simulink library "modularPlant_cl"  (R2018b)
settings: Solver=VariableStepAuto  StartTime=0.0  StopTime=10.0  RelTol=1e-3
undefined symbols (not defined in the file or in its folder): sim_param
libraries: animation_cl x1, fixedGroundStation_cl x1, tethers_cl x1, vehicle x1, winch_ul x1
settings Model: Creator=mcobb  LastModifiedBy=mcobb

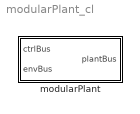
== system modularPlant_cl ==
  modularPlant : Subsystem  VariantControl=VSS_plant_modularPlant

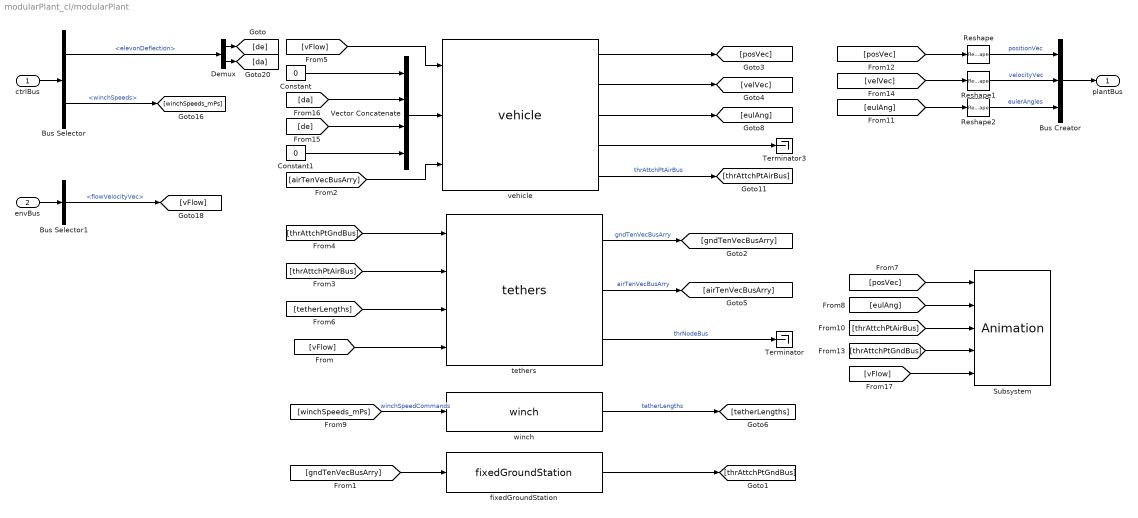
== system modularPlant_cl/modularPlant ==
  ctrlBus : Inport  OutDataTypeStr=Bus: ctrlBus
  envBus : Inport  Port=2  OutDataTypeStr=Bus: envBus
  Bus Creator : BusCreator  Inputs=3  OutDataTypeStr=Bus: plantBus
  Bus Selector : BusSelector  OutputSignals=elevonDeflection,winchSpeeds
  Bus Selector1 : BusSelector  OutputSignals=flowVelocityVec
  Constant : Constant  Value=0
  Constant1 : Constant  Value=0
  Demux : Demux  Outputs=2
  Reshape : Reshape  OutputDimensionality=Column vector (2-D)
  Reshape1 : Reshape  OutputDimensionality=Column vector (2-D)
  Reshape2 : Reshape  OutputDimensionality=Column vector (2-D)
  Subsystem : animation_cl/Animation  SystemSampleTime=-1
  Terminator : Terminator
  Terminator3 : Terminator
  Vector Concatenate : Concatenate  NumInputs=4
  fixedGroundStation : fixedGroundStation_cl/fixedGroundStation  fixed=1  J=sim_param.platform_param.platform_Izz  b=sim_param.platform_param.platform_damping  posVec=[0 0 0]  thr1AttachPt=sim_param.tether_imp_nodes.R11_g  thr2AttachPt=sim_param.tether_imp_nodes.R21_g  thr3AttachPt=sim_param.tether_imp_nodes.R31_g  initAngPos=ini_platform_ang  initAngVel=ini_platform_vel
  tethers : tethers_cl/tethers  thr=thr
  vehicle : vehicle/vehicle  SystemSampleTime=-1
  winch : winch_ul/winch  wnch=winch
  plantBus : Outport  OutDataTypeStr=Bus: plantBus
  wires:
  Bus Selector1/1 -> [vFlow]  "<flowVelocityVec>"
  envBus/1 -> Bus Selector1/1
  ctrlBus/1 -> Bus Selector/1
  Bus Selector/2 -> [winchSpeeds_mPs]  "<winchSpeeds>"
  Bus Creator/1 -> plantBus/1
  Reshape/1 -> Bus Creator/1  "positionVec"
  Reshape2/1 -> Bus Creator/3  "eulerAngles"
  Reshape1/1 -> Bus Creator/2  "velocityVec"
  winch/1 -> [tetherLengths]  "tetherLengths"
  [winchSpeeds_mPs] -> winch/1  "winchSpeedCommands"
  [posVec] -> Reshape/1
  [velVec] -> Reshape1/1
  [eulAng] -> Reshape2/1
  vehicle/3 -> [eulAng]
  vehicle/1 -> [posVec]
  vehicle/5 -> [thrAttchPtAirBus]  "thrAttchPtAirBus"
  vehicle/2 -> [velVec]
  vehicle/4 -> Terminator3/1
  [vFlow] -> vehicle/1
  Bus Selector/1 -> Demux/1  "<elevonDeflection>"
  Demux/2 -> [da]
  Demux/1 -> [de]
  [vFlow] -> tethers/4
  fixedGroundStation/1 -> [thrAttchPtGndBus]
  tethers/1 -> [gndTenVecBusArry]  "gndTenVecBusArry"
  tethers/2 -> [airTenVecBusArry]  "airTenVecBusArry"
  tethers/3 -> Terminator/1  "thrNodeBus"
  [gndTenVecBusArry] -> fixedGroundStation/1
  Constant/1 -> Vector Concatenate/1
  [da] -> Vector Concatenate/2
  [de] -> Vector Concatenate/3
  Constant1/1 -> Vector Concatenate/4
  [airTenVecBusArry] -> vehicle/3
  [thrAttchPtAirBus] -> tethers/2
  [thrAttchPtGndBus] -> tethers/1
  [tetherLengths] -> tethers/3
  [posVec] -> Subsystem/1
  [eulAng] -> Subsystem/2
  [thrAttchPtAirBus] -> Subsystem/3
  [thrAttchPtGndBus] -> Subsystem/4
  [vFlow] -> Subsystem/5
  Vector Concatenate/1 -> vehicle/2
